simulink model "lab1handson"  (R2020a)
settings: Solver=VariableStepAuto  StartTime=0.0  StopTime=10.0  RelTol=1e-3
PreLoadFcn:
  | a = -3;
  | b = -4;
  | Kp = 55;
  | Ki = 100;
  | m = 25;
  | t = [0:0.01:10]';
  | Ts = 0.01;
  | stin = [zeros(floor((length(t)/2)+1),1) ; 5*ones(floor(length(t)/2),1)];
  | itr = 200;
PostLoadFcn:
  | a = -3;
  | b = -4;
  | Kp = 55;
  | Ki = 100;
  | m = 25;
  | t = [0:0.01:10]';
  | Ts = 0.01;
  | stin = [zeros(floor((length(t)/2)+1),1) ; 5*ones(floor(length(t)/2),1)];
  | itr = 200;
settings Model: Creator=pawankumarf  LastModifiedBy=Jake
settings DataIOCC: ExternalInput=[t, stin]  LoadExternalInput=on  SaveFormat=Array  ReturnWorkspaceOutputs=off

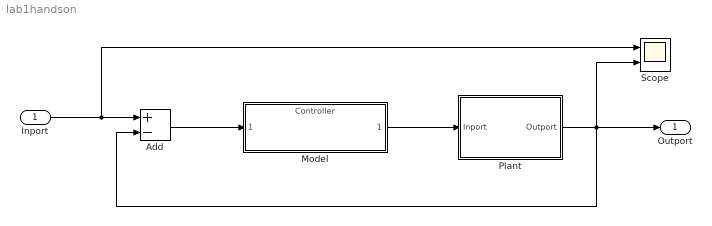
== system lab1handson ==
  Inport : Inport
  Add : Sum  Inputs=+-
  Model : ModelReference  ModelNameDialog=Controller.slx  ModelReferenceVersion=1.6
  Plant : Subsystem
  Scope : Scope  NumInputPorts=2
  Outport : Outport
  wires:
  Model/1 -> Plant/1(Inport)
  Plant/1(Outport) -> Scope/2, Outport/1, Add/2
  Inport/1 -> Scope/1, Add/1
  Add/1 -> Model/1

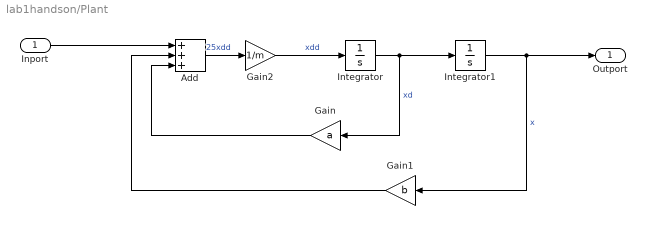
== system lab1handson/Plant ==
  Inport : Inport
  Add : Sum  Inputs=+++
  Gain : Gain  Gain=a
  Gain1 : Gain  Gain=b
  Gain2 : Gain  Gain=1/m
  Integrator : Integrator
  Integrator1 : Integrator
  Outport : Outport
  wires:
  Integrator/1 -> Integrator1/1, Gain/1  "xd"
  Gain1/1 -> Add/2
  Add/1 -> Gain2/1  "25xdd"
  Gain/1 -> Add/3
  Gain2/1 -> Integrator/1  "xdd"
  Integrator1/1 -> Outport/1, Gain1/1  "x"
  Inport/1 -> Add/1
